simulink model "UltrasonicDistanceSensor_4"  (R2023a)
settings: Solver=ode1  StartTime=0.0  StopTime=10.0  FixedStep=0.01  RelTol=1e-3
values from neighbouring files (symbols this model uses):
  max_range = 1    [init_sensor_params.m]
  min_range = 0.115    [init_sensor_params.m]
  quay_1_depth = 0    [init_sensor_params.m]
  quay_1_en = false    [init_sensor_params.m]
  quay_1_p0 = [0, 0]'    [init_sensor_params.m]
  quay_1_p1 = [0, 0]'    [init_sensor_params.m]
  quay_2_depth = 0    [init_sensor_params.m]
  quay_2_en = false    [init_sensor_params.m]
  quay_2_p0 = [0, 0]'    [init_sensor_params.m]
  quay_2_p1 = [0, 0]'    [init_sensor_params.m]
  quay_3_depth = 0    [init_sensor_params.m]
  quay_3_en = false    [init_sensor_params.m]
  quay_3_p0 = [0, 0]'    [init_sensor_params.m]
  quay_3_p1 = [0, 0]'    [init_sensor_params.m]
  quay_4_depth = 0    [init_sensor_params.m]
  quay_4_en = false    [init_sensor_params.m]
  quay_4_p0 = [0, 0]'    [init_sensor_params.m]
  quay_4_p1 = [0, 0]'    [init_sensor_params.m]
  sensor_pose_psi = 0    [init_sensor_params.m]
  sensor_pose_x = 0    [init_sensor_params.m]
  sensor_pose_y = 0    [init_sensor_params.m]
settings Model: Creator=MagneSirnes  LastModifiedBy=HalvorPlatou
settings DebuggingCC: UnconnectedInputMsg=warning  UnconnectedOutputMsg=warning  UnconnectedLineMsg=warning
settings ModelReferenceCC: EnableRefExpFcnMdlSchedulingChecks=on
settings RTWCC: DLArmComputeVersion=19.05

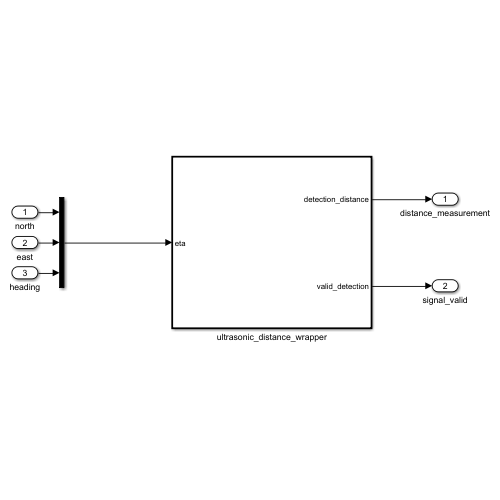
[thumbnail: Simulink's stored preview of the top-level diagram]
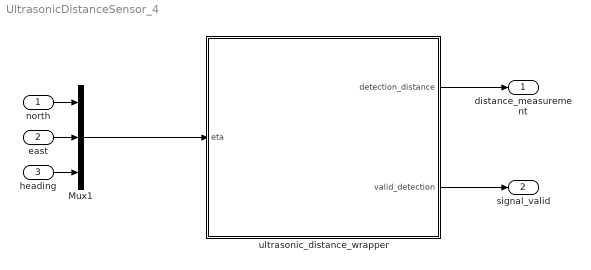
== system UltrasonicDistanceSensor_4 ==
  north : Inport  OutDataTypeStr=double
  east : Inport  Port=2  OutDataTypeStr=double
  heading : Inport  Port=3  OutDataTypeStr=double
  Mux1 : Mux  Inputs=3
  ultrasonic_distance_wrapper : MATLAB Function  TreatAsAtomicUnit=on
  distance_measurement : Outport  OutDataTypeStr=double  PortDimensions=1
  signal_valid : Outport  Port=2  OutDataTypeStr=boolean  PortDimensions=1
  wires:
  ultrasonic_distance_wrapper/2(valid_detection) -> signal_valid/1
  east/1 -> Mux1/2
  heading/1 -> Mux1/3
  north/1 -> Mux1/1
  ultrasonic_distance_wrapper/1(detection_distance) -> distance_measurement/1
  Mux1/1 -> ultrasonic_distance_wrapper/1(eta)

== matlab function UltrasonicDistanceSensor_4/ultrasonic_distance_wrapper ==
  data: eta input size=3; detection_distance output; valid_detection output; quay_1_en parameter; quay_1_depth parameter; quay_1_p1 parameter; quay_1_p0 parameter; quay_2_en parameter; quay_2_depth parameter; quay_2_p1 parameter; quay_2_p0 parameter; quay_3_en parameter; quay_3_depth parameter; quay_3_p1 parameter; quay_3_p0 parameter; quay_4_en parameter; quay_4_depth parameter; quay_4_p1 parameter; quay_4_p0 parameter; sensor_pose_x parameter; sensor_pose_y parameter; sensor_pose_psi parameter; min_range parameter; max_range parameter
function [detection_distance, valid_detection] = ultrasonic_distance_wrapper(eta, ... % 3dof ownship pose
    quay_1_en, quay_1_depth, quay_1_p1, quay_1_p0, quay_2_en, quay_2_depth, quay_2_p1, quay_2_p0, quay_3_en, quay_3_depth, quay_3_p1, quay_3_p0, quay_4_en, quay_4_depth, quay_4_p1, quay_4_p0, ... % quay parameters
    sensor_pose_x, sensor_pose_y, sensor_pose_psi, min_range, max_range) % sensor range and sensor pose in body frame

% ultrasonic_distance_wrapper - Wrapper for function ultrasonic_sensor()
%
% this handles accepting/parsing parameters from matlab workspace:
% quay, range, T_s_b 
% 
% ultrasonic_sensor() is wrapped in this way to ensure that its code
% remains visible and therefore maintainable and not hidden behind a
% simulink block. 

% Construct sensor to body transform
T_s_b = [
    cos(sensor_pose_psi), -sin(sensor_pose_psi), sensor_pose_x;
    sin(sensor_pose_psi),  cos(sensor_pose_psi), sensor_pose_y;
                       0,                     0,              1
];

% Construct quay parameters
num_quays = sum([quay_1_en, quay_2_en, quay_3_en, quay_4_en]);
s = struct('line', {nan(2, 2)}, 'depth', {nan});
quays = repmat(s,1,num_quays);

i = 1;

if quay_1_en
    quays(i).line = [reshape(quay_1_p0,2,1), reshape(quay_1_p1,2,1)];
    quays(i).depth = quay_1_depth;
    i = i+1;
end
if quay_2_en
    quays(i).line = [reshape(quay_2_p0,2,1), reshape(quay_2_p1,2,1)];
    quays(i).depth = quay_2_depth;
    i = i+1;
end
if quay_3_en
    quays(i).line = [reshape(quay_3_p0,2,1), reshape(quay_3_p1,2,1)];
    quays(i).depth = quay_3_depth;
    i = i+1;
end
if quay_4_en
    quays(i).line = [reshape(quay_4_p0,2,1), reshape(quay_4_p1,2,1)];
    quays(i).depth = quay_4_depth;
    i = i+1;
end

% Dispatch measurement generator
[dist, valid] = ultrasonic_sensor(eta, [min_range; max_range], quays, T_s_b);
% [detection_distance, valid_detection] = ultrasonic_sensor(eta, range, quays, T_s_b);

% simulink struggles to infer dimensions from calls to other matlab functions
% so selecting index (1,1) helps simulink realise that the return value is
% in fact a scalar.
detection_distance = dist(1,1);
valid_detection = valid(1,1);
